simulink library "tp264967"  (Simulink 3.0)
settings Model: LastModifiedBy=mato

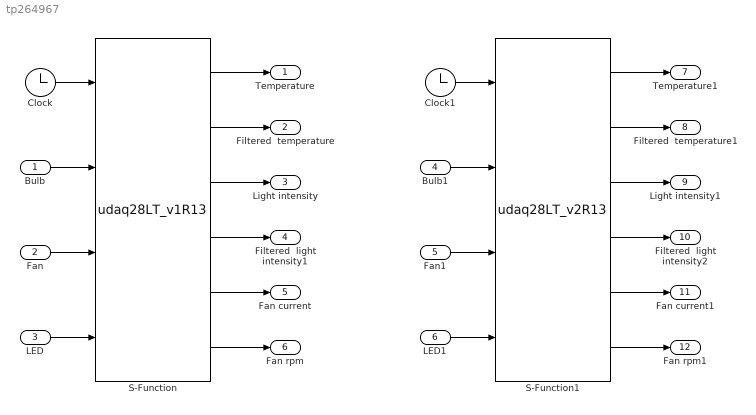
== system tp264967 ==
  Bulb : Inport  Port=1  PortWidth=-1  SampleTime=-1  DataType=auto
      settings: SignalType=auto
  Fan : Inport  Port=2  PortWidth=-1  SampleTime=-1  DataType=auto
      settings: SignalType=auto
  LED : Inport  Port=3  PortWidth=-1  SampleTime=-1  DataType=auto
      settings: SignalType=auto
  Bulb1 : Inport  Port=4  PortWidth=-1  SampleTime=-1  DataType=auto
      settings: SignalType=auto
  Fan1 : Inport  Port=5  PortWidth=-1  SampleTime=-1  DataType=auto
      settings: SignalType=auto
  LED1 : Inport  Port=6  PortWidth=-1  SampleTime=-1  DataType=auto
      settings: SignalType=auto
  Clock : Clock
      settings: DisplayTime=off  Decimation=10
  Clock1 : Clock
      settings: DisplayTime=off  Decimation=10
  S-Function : S-Function  Priority=1  FunctionName=udaq28LT_v1R13  Parameters=com_port, Ts, events_ot, rd_timeout, matlab_prior, warning, printout  PortCounts=[]  SFunctionModules=''  mask(uDAQ28/LT Communication Interface){com_port=COM3, Ts=0.5, events_ot=2, rd_timeout=80, matlab_prior=ABOVE_NORMAL_PRIORITY, warning=on, printout=off}
      mask prompts: com_port "Serial port:"; Ts "Sample time (sec):"; events_ot "Sampling delayed (%):"; rd_timeout "Read timeout (msec, lower than sample time):"; matlab_prior "Matlab priority"; warning "Warning if delayed (error if unchecked)"; printout "Detailed timing and timeout  printout"
      mask help:
      | (c) 2006 Martin Kamensky
      |
      | Serial port - USB serial port number assigned to uDAQ28/LT system
      |
      | Sampling time (sec) - the lowest working value in Windows is about 0.04 - 0.05 s
      |
      | Sample delayed (%) - number of events (percentually) when simulink loop can take more than time determined by sample time
      |
      | Read timeout (msec) - timeout for reading data from the port (the lowest working value is about 25 ms)
      |
      | Matlab priority :
      | NORMAL_PRIORITY - priority of common Windows application
      | ABOVE_NORMAL_PRIORITY - recommended - higher priority than common Windows application priority
      | HIGH_PRIORITY - recommended - high priority
      | REALTIME_PRIORITY - NOT recommended - takes almost all system resources
      mask init:
      | set_param(bdroot,'FixedStep',get_param(gcb,'Ts'));
      | set_param(bdroot,'Solver','ode1');
      | set_param(bdroot,'SolverMode','SingleTasking');
      | more off;
      mask StyleString: popup(COM1|COM2|COM3|COM4),edit,edit,edit,popup(NORMAL_PRIORITY|ABOVE_NORMAL_PRIORITY|HIGH_PRIORITY|REALTIME_PRIORITY),checkbox,checkbox
      mask CallbackString:
      | |set_param(bdroot,'FixedStep',get_param(gcb,'Ts'));
      | set_param(bdroot,'Solver','ode1');
      | set_param(bdroot,'SolverMode','SingleTasking');|||||
  S-Function1 : S-Function  Priority=1  FunctionName=udaq28LT_v2R13  Parameters=com_port, Ts, events_ot, rd_timeout, matlab_prior, warning, printout  PortCounts=[]  SFunctionModules=''  mask(uDAQ28/LT Communication Interface){com_port=COM3, Ts=0.5, events_ot=2, rd_timeout=80, matlab_prior=ABOVE_NORMAL_PRIORITY, warning=on, printout=on}
      mask prompts: com_port "Serial port:"; Ts "Sample time (sec):"; events_ot "Sampling delayed (%):"; rd_timeout "Read timeout (msec, lower than sample time):"; matlab_prior "Matlab priority"; warning "Warning if delayed (error if unchecked)"; printout "Detailed timing and timeout  printout"
      mask help:
      | (c) 2006 Martin Kamensky
      |
      | Serial port - USB serial port number assigned to uDAQ28/LT system
      |
      | Sampling time (sec) - the lowest working value in Windows is about 0.04 - 0.05 s
      |
      | Sample delayed (%) - number of events (percentually) when simulink loop can take more than time determined by sample time
      |
      | Read timeout (msec) - timeout for reading data from the port (the lowest working value is about 25 ms)
      |
      | Matlab priority :
      | NORMAL_PRIORITY - priority of common Windows application
      | ABOVE_NORMAL_PRIORITY - recommended - higher priority than common Windows application priority
      | HIGH_PRIORITY - recommended - high priority
      | REALTIME_PRIORITY - NOT recommended - takes almost all system resources
      mask init:
      | set_param(bdroot,'FixedStep',get_param(gcb,'Ts'));
      | set_param(bdroot,'Solver','ode1');
      | set_param(bdroot,'SolverMode','SingleTasking');
      | more off;
      mask StyleString: popup(COM1|COM2|COM3|COM4),edit,edit,edit,popup(NORMAL_PRIORITY|ABOVE_NORMAL_PRIORITY|HIGH_PRIORITY|REALTIME_PRIORITY),checkbox,checkbox
      mask CallbackString:
      | |set_param(bdroot,'FixedStep',get_param(gcb,'Ts'));
      | set_param(bdroot,'Solver','ode1');
      | set_param(bdroot,'SolverMode','SingleTasking');|||||
  Temperature : Outport  Port=1
  Filtered  temperature : Outport  Port=2
  Light intensity : Outport  Port=3
  Filtered  light intensity1 : Outport  Port=4
  Fan current : Outport  Port=5
  Fan rpm : Outport  Port=6
  Temperature1 : Outport  Port=7
  Filtered  temperature1 : Outport  Port=8
  Light intensity1 : Outport  Port=9
  Filtered  light intensity2 : Outport  Port=10
  Fan current1 : Outport  Port=11
  Fan rpm1 : Outport  Port=12
  wires:
  S-Function/1 -> Temperature/1
  S-Function/2 -> Filtered  temperature/1
  Clock/1 -> S-Function/1
  Bulb/1 -> S-Function/2
  Fan/1 -> S-Function/3
  S-Function/3 -> Light intensity/1
  S-Function/4 -> Filtered  light intensity1/1
  S-Function/5 -> Fan current/1
  S-Function/6 -> Fan rpm/1
  LED/1 -> S-Function/4
  S-Function1/1 -> Temperature1/1
  S-Function1/2 -> Filtered  temperature1/1
  Clock1/1 -> S-Function1/1
  Bulb1/1 -> S-Function1/2
  Fan1/1 -> S-Function1/3
  S-Function1/3 -> Light intensity1/1
  S-Function1/4 -> Filtered  light intensity2/1
  S-Function1/5 -> Fan current1/1
  S-Function1/6 -> Fan rpm1/1
  LED1/1 -> S-Function1/4
